simulink model "IMU_board_example_IMU_grouped"  (R2015b)
settings: Solver=ode1  StartTime=0.0  StopTime=inf  FixedStep=.0005  RelTol=1e-3
undefined symbols (not defined in the file or in its folder): deg, s
libraries: qbmove_library_2015b x1, QB_pacer_lib x1, qbmove_library x1
settings Model: Creator=laurentio  LastModifiedBy=MattiaCP
settings DataIOCC: SaveFormat=Array
settings DebuggingCC: UnderspecifiedInitializationDetection=Classic  MergeDetectMultiDrivingBlocksExec=none  SolverPrmCheckMsg=warning  StateNameClashWarn=warning
settings HardwareCC: ProdBitPerPointer=32  ProdLargestAtomicFloat=None  ProdIntDivRoundTo=Undefined  ProdEndianess=Unspecified  ProdWordSize=32  ProdHWDeviceType=32-bit Generic
settings GRTTargetCC: GeneratePreprocessorConditionals=Disable all
settings ConfigComp: CovModelRefEnable=Off  CovSFcnEnable=off

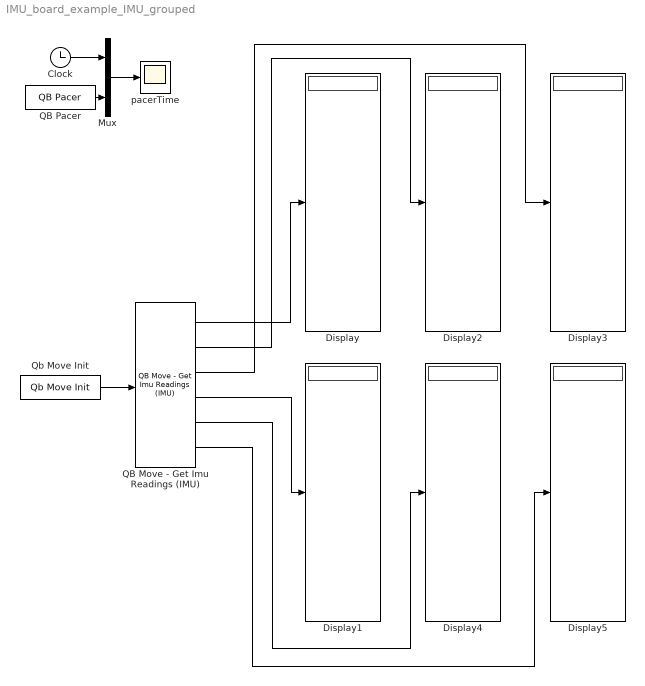
== system IMU_board_example_IMU_grouped ==
  Clock : Clock
  Display{,1..5} (6 alike) : Display
  Mux : Mux  Inputs=2
  QB Move - Get Imu Readings (IMU) : qbmove_library_2015b/QB Move - Get Imu Readings (IMU)  ID=1  N_IMU=6  DAISY_CHAINING=off  ACC_UNITY=G  GYRO_UNITY=deg/s  MAG_UNITY=uT
  QB Pacer : QB_pacer_lib/QB Pacer  simTimePerRealTime=1
  Qb Move Init : qbmove_library/Qb Move Init  NUMBER_OF_COM='COM2'  BAUD_RATE_COM=2000000
  pacerTime : Scope
  wires:
  QB Pacer/1 -> Mux/2
  Clock/1 -> Mux/1
  Qb Move Init/1 -> QB Move - Get Imu Readings (IMU)/1
  Mux/1 -> pacerTime/1
  QB Move - Get Imu Readings (IMU)/1 -> Display/1
  QB Move - Get Imu Readings (IMU)/2 -> Display2/1
  QB Move - Get Imu Readings (IMU)/3 -> Display3/1
  QB Move - Get Imu Readings (IMU)/4 -> Display1/1
  QB Move - Get Imu Readings (IMU)/5 -> Display4/1
  QB Move - Get Imu Readings (IMU)/6 -> Display5/1
